simulink model "sistema"  (R2023a)
settings: Solver=VariableStepAuto  StartTime=0.0  StopTime=100.0  RelTol=1e-3
settings Model: Creator=Usuario  LastModifiedBy=Usuario
settings DataIOCC: ReturnWorkspaceOutputs=off  TimeSaveName=t

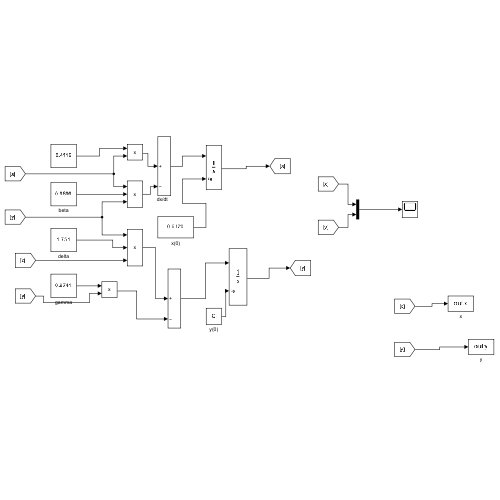
[thumbnail: Simulink's stored preview of the top-level diagram]
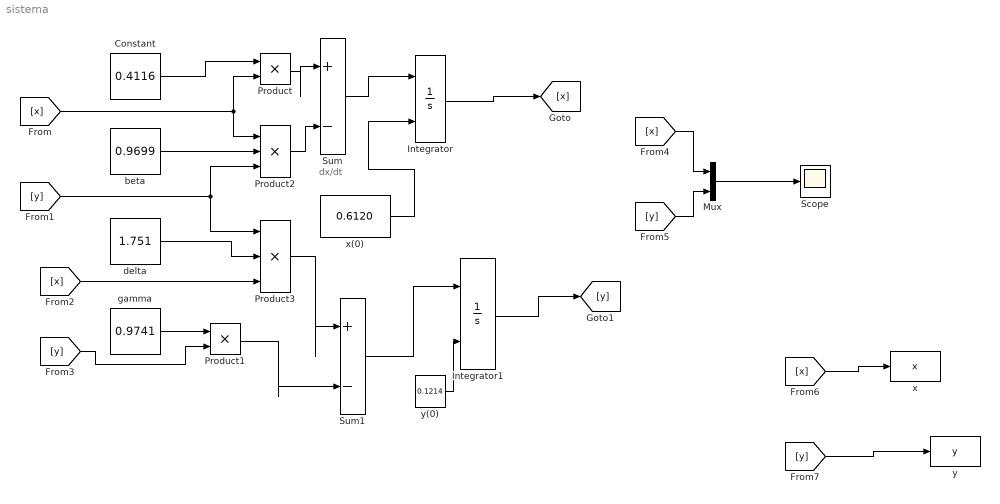
== system sistema ==
  note: dx/dt
  Constant : Constant  Value=0.4116
  Integrator : Integrator  InitialConditionSource=external
  Integrator1 : Integrator  InitialConditionSource=external
  Mux : Mux  Inputs=2
  Product : Product
  Product1 : Product
  Product2 : Product  Inputs=3
  Product3 : Product  Inputs=3
  Scope : Scope
  Sum : Sum  Inputs=|+-
  Sum1 : Sum  Inputs=|+-
  beta : Constant  Value=0.9699
  delta : Constant  Value=1.751
  gamma : Constant  Value=0.9741
  x : ToWorkspace  VariableName=x  SampleTime=-1
  x(0) : Constant  Value=0.6120
  y : ToWorkspace  VariableName=y  SampleTime=-1
  y(0) : Constant  Value=0.1214
  wires:
  Constant/1 -> Product/1
  [x] -> Product2/1, Product/2
  Product/1 -> Sum/1
  Product2/1 -> Sum/2
  beta/1 -> Product2/2
  [y] -> Product3/1, Product2/3
  delta/1 -> Product3/2
  [x] -> Product3/3
  gamma/1 -> Product1/1
  [y] -> Product1/2
  Sum/1 -> Integrator/1
  x(0)/1 -> Integrator/2
  Product3/1 -> Sum1/1
  Product1/1 -> Sum1/2
  Sum1/1 -> Integrator1/1
  y(0)/1 -> Integrator1/2
  Integrator/1 -> [x]
  Integrator1/1 -> [y]
  Mux/1 -> Scope/1
  [x] -> Mux/1
  [y] -> Mux/2
  [x] -> x/1
  [y] -> y/1
